simulink model "ackerman_ROS_neural_controller_v2"  (R2023a)
settings: Solver=FixedStepDiscrete  StartTime=0.0  StopTime=200  FixedStep=0.1  RelTol=1e-3
undefined symbols (not defined in the file or in its folder): Angular, Linear
libraries: neural x413, robotlib x15, robotcorelib x1
(part 10 of 17)

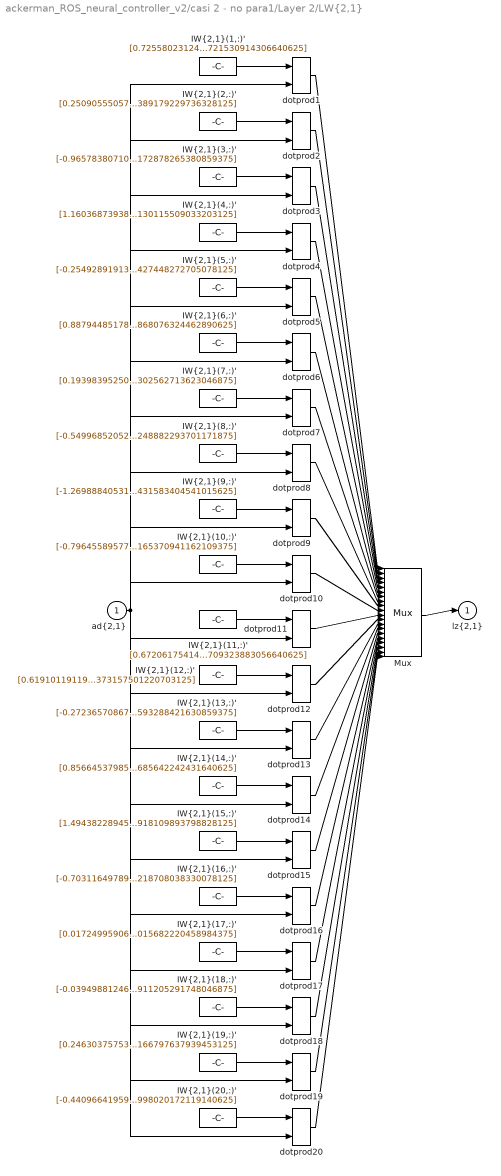
== system ackerman_ROS_neural_controller_v2/casi 2 - no para1/Layer 2/LW{2,1} ==
  "ad{2,1}" : Inport  PortDimensions=10  SampleTime=0.1
      mask Display: e = 0.06;c1 = [120 230 180]/255;c2 = ([120 230 180]+0)/(256+128);c3 = ([120 230 180]+128)/(256+128);patch([0 1 1 0],[0 0 1 1],c1);patch([0 1 1 1-e 1-e 0+e],[0 0 1 1-e 0+e 0+e],c2);patch([0 0 1 1-e 0+e 0+e],[0 1 1 1-e 1-e 0+e],c3);plot([0 1 1 0 0],[0 0 1 1 0]);
  "IW{2,1}(1,:)'" : Constant  Value=[0.7255802312437111822873703204095363616943359375;-0.959135021271336984938216119189746677875518798828125;0.292195933309013111678353880051872693002223968505859375;1.3155053067483366557866020229994319379329681396484375;-0.851881968454604621143744225264526903629302978515625;-1.0328524281587456723485729526146315038204193115234375;-0.2725914664811670551358702141442336142063140869140625;0.69933961328985816408021491952240467071533203125;-0.088878783625517987498909633359289728105068206787109375;-0.4504789263447295244446877404698170721530914306640625]
      mask Display: e = 0.06;c1 = [120 150 230]/255;c2 = ([120 150 230]+0)/383;c3 = ([120 150 230]+128)/383;patch([0 1 1 0],[0 0 1 1],c1);patch([0 1 1 1-e 1-e 0+e],[0 0 1 1-e 0+e 0+e],c2);patch([0 0 1 1-e 0+e 0+e],[0 1 1 1-e 1-e 0+e],c3);plot([0 1 1 0 0],[0 0 1 1 0]);disp('weights');
  "IW{2,1}(10,:)'" : Constant  Value=[-0.79645589577707454065347292271326296031475067138671875;0.255979770260327421649293455629958771169185638427734375;-0.258539951097875475571896686233230866491794586181640625;1.0207788991495245767282540327869355678558349609375;-0.24124933524105329762932115045259706676006317138671875;-0.72258293758172931209315947853610850870609283447265625;0.87006263229923608282234681610134430229663848876953125;-0.70559758504935310430283834648435004055500030517578125;-0.0123525145129407022681622407844770350493490695953369140625;-0.6747862752605688907436842782772146165370941162109375]
      mask Display: e = 0.06;c1 = [120 150 230]/255;c2 = ([120 150 230]+0)/383;c3 = ([120 150 230]+128)/383;patch([0 1 1 0],[0 0 1 1],c1);patch([0 1 1 1-e 1-e 0+e],[0 0 1 1-e 0+e 0+e],c2);patch([0 0 1 1-e 0+e 0+e],[0 1 1 1-e 1-e 0+e],c3);plot([0 1 1 0 0],[0 0 1 1 0]);disp('weights');
  "IW{2,1}(11,:)'" : Constant  Value=[0.67206175414446589488903782694251276552677154541015625;0.425012143990661284131959973819903098046779632568359375;-0.90070904319052724762428852045559324324131011962890625;-0.71047514245276188749045331860543228685855865478515625;0.62743503657371579862456201226450502872467041015625;-0.40397353982891914814246092646499164402484893798828125;0.1265477401734184381698611332467407919466495513916015625;-0.416411569496611011498288235088693909347057342529296875;0.0269578242680961095711911212902123224921524524688720703125;1.9286984680039014339314462631591595709323883056640625]
      mask Display: e = 0.06;c1 = [120 150 230]/255;c2 = ([120 150 230]+0)/383;c3 = ([120 150 230]+128)/383;patch([0 1 1 0],[0 0 1 1],c1);patch([0 1 1 1-e 1-e 0+e],[0 0 1 1-e 0+e 0+e],c2);patch([0 0 1 1-e 0+e 0+e],[0 1 1 1-e 1-e 0+e],c3);plot([0 1 1 0 0],[0 0 1 1 0]);disp('weights');
  "IW{2,1}(12,:)'" : Constant  Value=[0.61910119119551865196626749821007251739501953125;1.5566506758364762053048480083816684782505035400390625;0.007559785691830124727819129049066759762354195117950439453125;-0.2271652971788542807463073813778464682400226593017578125;-1.03507488578625395092558392207138240337371826171875;0.218995547321044925492827815105556510388851165771484375;0.257413353310532999618231997374095954000949859619140625;-0.09074896375455325514547411103194463066756725311279296875;0.51244231388938688009915267684846185147762298583984375;0.69550664112394511295889287794125266373157501220703125]
      mask Display: e = 0.06;c1 = [120 150 230]/255;c2 = ([120 150 230]+0)/383;c3 = ([120 150 230]+128)/383;patch([0 1 1 0],[0 0 1 1],c1);patch([0 1 1 1-e 1-e 0+e],[0 0 1 1-e 0+e 0+e],c2);patch([0 0 1 1-e 0+e 0+e],[0 1 1 1-e 1-e 0+e],c3);plot([0 1 1 0 0],[0 0 1 1 0]);disp('weights');
  "IW{2,1}(13,:)'" : Constant  Value=[-0.2723657086743267452533245887025259435176849365234375;0.51216475864015154062514056931831873953342437744140625;-1.0193552597301509532456975648528896272182464599609375;-1.1847191291297889392808428965508937835693359375;1.0773368660683753095241854680352844297885894775390625;0.0962534189837907228071145482317660935223102569580078125;-0.417721772937184265828136631171219050884246826171875;0.38947970915216412191028894085320644080638885498046875;0.337210418509659159980174081283621490001678466796875;0.220079813772727062026746125411591492593288421630859375]
      mask Display: e = 0.06;c1 = [120 150 230]/255;c2 = ([120 150 230]+0)/383;c3 = ([120 150 230]+128)/383;patch([0 1 1 0],[0 0 1 1],c1);patch([0 1 1 1-e 1-e 0+e],[0 0 1 1-e 0+e 0+e],c2);patch([0 0 1 1-e 0+e 0+e],[0 1 1 1-e 1-e 0+e],c3);plot([0 1 1 0 0],[0 0 1 1 0]);disp('weights');
  "IW{2,1}(14,:)'" : Constant  Value=[0.85664537985749278359293157336651347577571868896484375;0.56640828026000511474791210275725461542606353759765625;0.0140221107131337473228338552644345327280461788177490234375;0.2148298691543548966098597929885727353394031524658203125;-0.93403619601038467834541734191589057445526123046875;0.12856379595534705995163449188112281262874603271484375;-0.75467959982227217352601655875332653522491455078125;-0.63322516283317298313448873159359209239482879638671875;-1.0672216572169812565107349655590951442718505859375;-0.6144516641324175854066425017663277685642242431640625]
      mask Display: e = 0.06;c1 = [120 150 230]/255;c2 = ([120 150 230]+0)/383;c3 = ([120 150 230]+128)/383;patch([0 1 1 0],[0 0 1 1],c1);patch([0 1 1 1-e 1-e 0+e],[0 0 1 1-e 0+e 0+e],c2);patch([0 0 1 1-e 0+e 0+e],[0 1 1 1-e 1-e 0+e],c3);plot([0 1 1 0 0],[0 0 1 1 0]);disp('weights');
  "IW{2,1}(15,:)'" : Constant  Value=[1.494382289455435941505356822744943201541900634765625;-0.38028619508781480451631296091363765299320220947265625;-1.0111267060786659488513805627007968723773956298828125;-0.488055297640631380318154697306454181671142578125;0.3434831730449758868672915923525579273700714111328125;1.216268037924192579879445474944077432155609130859375;-0.1970804861360637982858889927229029126465320587158203125;-0.30493588644459268532926898842561058700084686279296875;1.429852600353733738103301220689900219440460205078125;0.55184388765904046625365708678145892918109893798828125]
      mask Display: e = 0.06;c1 = [120 150 230]/255;c2 = ([120 150 230]+0)/383;c3 = ([120 150 230]+128)/383;patch([0 1 1 0],[0 0 1 1],c1);patch([0 1 1 1-e 1-e 0+e],[0 0 1 1-e 0+e 0+e],c2);patch([0 0 1 1-e 0+e 0+e],[0 1 1 1-e 1-e 0+e],c3);plot([0 1 1 0 0],[0 0 1 1 0]);disp('weights');
  "IW{2,1}(16,:)'" : Constant  Value=[-0.70311649789439478741570610509370453655719757080078125;0.82719449320928128965846326536848209798336029052734375;0.52011078229624552182741581418667919933795928955078125;-0.7482339633582888449581105305696837604045867919921875;0.260733776152210439125411767236073501408100128173828125;1.257014055969282839697598319617100059986114501953125;0.514007980751157500520776011398993432521820068359375;0.06832775328143329829355678839419852010905742645263671875;1.355094864178037372681728811585344374179840087890625;0.58915716345959900923645591319655068218708038330078125]
      mask Display: e = 0.06;c1 = [120 150 230]/255;c2 = ([120 150 230]+0)/383;c3 = ([120 150 230]+128)/383;patch([0 1 1 0],[0 0 1 1],c1);patch([0 1 1 1-e 1-e 0+e],[0 0 1 1-e 0+e 0+e],c2);patch([0 0 1 1-e 0+e 0+e],[0 1 1 1-e 1-e 0+e],c3);plot([0 1 1 0 0],[0 0 1 1 0]);disp('weights');
  "IW{2,1}(17,:)'" : Constant  Value=[0.01724995906974446935322475837892852723598480224609375;-0.87370370646173001194512153233517892658710479736328125;1.02449594010034417124188621528446674346923828125;0.3546780425879723086524109021411277353763580322265625;0.5542510541573941740267628119909204542636871337890625;-1.519879697911841187618620097055099904537200927734375;1.9952410695173907750898933954886160790920257568359375;0.522496701742714453331473123398609459400177001953125;0.60216071280023564238348399157985113561153411865234375;1.3489645232526699114572465987293981015682220458984375]
      mask Display: e = 0.06;c1 = [120 150 230]/255;c2 = ([120 150 230]+0)/383;c3 = ([120 150 230]+128)/383;patch([0 1 1 0],[0 0 1 1],c1);patch([0 1 1 1-e 1-e 0+e],[0 0 1 1-e 0+e 0+e],c2);patch([0 0 1 1-e 0+e 0+e],[0 1 1 1-e 1-e 0+e],c3);plot([0 1 1 0 0],[0 0 1 1 0]);disp('weights');
  "IW{2,1}(18,:)'" : Constant  Value=[-0.039498812461870889956028207734561874531209468841552734375;0.458104116462539512344420700173941440880298614501953125;-0.12868703006185155945928499932051636278629302978515625;0.68295350186009751158877634225063957273960113525390625;-1.0871944340971875231360854741069488227367401123046875;-0.42803001209135571603070502533228136599063873291015625;0.012944291652409345427798825767240487039089202880859375;0.8094050995384247659814036524039693176746368408203125;-0.562292589961300048884140778682194650173187255859375;0.1292007200127660293542675162825617007911205291748046875]
      mask Display: e = 0.06;c1 = [120 150 230]/255;c2 = ([120 150 230]+0)/383;c3 = ([120 150 230]+128)/383;patch([0 1 1 0],[0 0 1 1],c1);patch([0 1 1 1-e 1-e 0+e],[0 0 1 1-e 0+e 0+e],c2);patch([0 0 1 1-e 0+e 0+e],[0 1 1 1-e 1-e 0+e],c3);plot([0 1 1 0 0],[0 0 1 1 0]);disp('weights');
  "IW{2,1}(19,:)'" : Constant  Value=[0.2463037575343004770278554360629641450941562652587890625;1.082908833346408528086612932384014129638671875;-0.5431543815046693257642118624062277376651763916015625;1.2737764365786403697455853034625761210918426513671875;0.543977471682644431183462074841372668743133544921875;-0.85893985210927337181630036866408772766590118408203125;1.871626995457029263292270115925930440425872802734375;0.0825784829680522580730439585749991238117218017578125;-1.654760344583033226939505766495130956172943115234375;0.2404324935540936014621848926253733225166797637939453125]
      mask Display: e = 0.06;c1 = [120 150 230]/255;c2 = ([120 150 230]+0)/383;c3 = ([120 150 230]+128)/383;patch([0 1 1 0],[0 0 1 1],c1);patch([0 1 1 1-e 1-e 0+e],[0 0 1 1-e 0+e 0+e],c2);patch([0 0 1 1-e 0+e 0+e],[0 1 1 1-e 1-e 0+e],c3);plot([0 1 1 0 0],[0 0 1 1 0]);disp('weights');
  "IW{2,1}(2,:)'" : Constant  Value=[0.2509055505702744159890471564722247421741485595703125;-1.25881579798349463317208574153482913970947265625;1.33862512869737404486158993677236139774322509765625;0.315714701756230564644312153177452273666858673095703125;-1.2366679233488728772982767623034305870532989501953125;0.3493751303882339787065802738652564585208892822265625;0.01409598964836229935404521285136070218868553638458251953125;1.27609628826768695120108532137237489223480224609375;-0.1335788420752038463401589751811116002500057220458984375;-0.93661901416684145704749653305043466389179229736328125]
      mask Display: e = 0.06;c1 = [120 150 230]/255;c2 = ([120 150 230]+0)/383;c3 = ([120 150 230]+128)/383;patch([0 1 1 0],[0 0 1 1],c1);patch([0 1 1 1-e 1-e 0+e],[0 0 1 1-e 0+e 0+e],c2);patch([0 0 1 1-e 0+e 0+e],[0 1 1 1-e 1-e 0+e],c3);plot([0 1 1 0 0],[0 0 1 1 0]);disp('weights');
  "IW{2,1}(20,:)'" : Constant  Value=[-0.44096641959653981590605553719797171652317047119140625;0.7083902543346669578028240721323527395725250244140625;-0.5166341286167612789625991354114376008510589599609375;0.9049323980779118148376483077299781143665313720703125;-1.271794249096482420924303369247354567050933837890625;-0.68138595653020306297520392035949043929576873779296875;-0.90212325864638021055696981420624069869518280029296875;-0.45820526458276022996329857051023282110691070556640625;-0.020846715917271947671185472472643596120178699493408203125;-0.68369139124353583980564508237875998020172119140625]
      mask Display: e = 0.06;c1 = [120 150 230]/255;c2 = ([120 150 230]+0)/383;c3 = ([120 150 230]+128)/383;patch([0 1 1 0],[0 0 1 1],c1);patch([0 1 1 1-e 1-e 0+e],[0 0 1 1-e 0+e 0+e],c2);patch([0 0 1 1-e 0+e 0+e],[0 1 1 1-e 1-e 0+e],c3);plot([0 1 1 0 0],[0 0 1 1 0]);disp('weights');
  "IW{2,1}(3,:)'" : Constant  Value=[-0.9657838071053219675121681575546972453594207763671875;-0.29459222518749650365776915350579656660556793212890625;-0.9657645759044359845546523501980118453502655029296875;0.472664168879096069364464938189485110342502593994140625;-0.4647204412011516350133888408890925347805023193359375;0.0489842324695661524014411725147510878741741180419921875;-0.470447392631997807210808559830184094607830047607421875;-0.75556461890030190975409141174168325960636138916015625;-0.77960517042681154453731551257078535854816436767578125;0.1635230428322337059565683148321113549172878265380859375]
      mask Display: e = 0.06;c1 = [120 150 230]/255;c2 = ([120 150 230]+0)/383;c3 = ([120 150 230]+128)/383;patch([0 1 1 0],[0 0 1 1],c1);patch([0 1 1 1-e 1-e 0+e],[0 0 1 1-e 0+e 0+e],c2);patch([0 0 1 1-e 0+e 0+e],[0 1 1 1-e 1-e 0+e],c3);plot([0 1 1 0 0],[0 0 1 1 0]);disp('weights');
  "IW{2,1}(4,:)'" : Constant  Value=[1.1603687393829453800009332553599961102008819580078125;-0.43444035743057363152530570005183108150959014892578125;-0.2327820794505396639895167254508123733103275299072265625;1.0752460303334367974770202636136673390865325927734375;0.0409481506539224049401326510633225552737712860107421875;-0.52422297129341666188651061020209453999996185302734375;0.97732432532743407360698029151535592973232269287109375;1.670364407889719959854346598149277269840240478515625;-0.57438837959386257470129066859954036772251129150390625;0.06045821031614935503473162725640577264130115509033203125]
      mask Display: e = 0.06;c1 = [120 150 230]/255;c2 = ([120 150 230]+0)/383;c3 = ([120 150 230]+128)/383;patch([0 1 1 0],[0 0 1 1],c1);patch([0 1 1 1-e 1-e 0+e],[0 0 1 1-e 0+e 0+e],c2);patch([0 0 1 1-e 0+e 0+e],[0 1 1 1-e 1-e 0+e],c3);plot([0 1 1 0 0],[0 0 1 1 0]);disp('weights');
  "IW{2,1}(5,:)'" : Constant  Value=[-0.254928919131068576486853771712048910558223724365234375;0.73622325216995931906893702034722082316875457763671875;-0.2115569379132722083181050720668281428515911102294921875;0.16011668696643288622993850367492996156215667724609375;-1.007294432717205978633501217700541019439697265625;0.879084198460805765762415830977261066436767578125;0.57105308322778036700384518553619273006916046142578125;-0.1648122755865679411879654026051866821944713592529296875;0.9415158413094939504617286729626357555389404296875;0.525759644457871377909441434894688427448272705078125]
      mask Display: e = 0.06;c1 = [120 150 230]/255;c2 = ([120 150 230]+0)/383;c3 = ([120 150 230]+128)/383;patch([0 1 1 0],[0 0 1 1],c1);patch([0 1 1 1-e 1-e 0+e],[0 0 1 1-e 0+e 0+e],c2);patch([0 0 1 1-e 0+e 0+e],[0 1 1 1-e 1-e 0+e],c3);plot([0 1 1 0 0],[0 0 1 1 0]);disp('weights');
  "IW{2,1}(6,:)'" : Constant  Value=[0.88794485178955573356773811610764823853969573974609375;0.2324274258381906488324375459342263638973236083984375;0.858625944853660172384479665197432041168212890625;-0.79953285474529989240721761234453879296779632568359375;0.3246840807043895882344486381043680012226104736328125;0.70300148951327512403253194861463271081447601318359375;0.72709749834294801207335012804833240807056427001953125;-0.059841883781344189230377850208242307417094707489013671875;0.55259353871622185483403200123575516045093536376953125;0.303105422786621725439459851259016431868076324462890625]
      mask Display: e = 0.06;c1 = [120 150 230]/255;c2 = ([120 150 230]+0)/383;c3 = ([120 150 230]+128)/383;patch([0 1 1 0],[0 0 1 1],c1);patch([0 1 1 1-e 1-e 0+e],[0 0 1 1-e 0+e 0+e],c2);patch([0 0 1 1-e 0+e 0+e],[0 1 1 1-e 1-e 0+e],c3);plot([0 1 1 0 0],[0 0 1 1 0]);disp('weights');
  "IW{2,1}(7,:)'" : Constant  Value=[0.19398395250211120099947947892360389232635498046875;0.1806780802861871204623156472734990529716014862060546875;1.06574239323498431986081413924694061279296875;-0.17040549486612699414678218090557493269443511962890625;0.89158393834403704136803980873082764446735382080078125;-1.4919986389830948159129775376641191542148590087890625;-0.69437571656851115875497271190397441387176513671875;0.75295094637079718058458865925786085426807403564453125;-0.8595816234580855308422542293556034564971923828125;0.384089854587841894595356961872312240302562713623046875]
      mask Display: e = 0.06;c1 = [120 150 230]/255;c2 = ([120 150 230]+0)/383;c3 = ([120 150 230]+128)/383;patch([0 1 1 0],[0 0 1 1],c1);patch([0 1 1 1-e 1-e 0+e],[0 0 1 1-e 0+e 0+e],c2);patch([0 0 1 1-e 0+e 0+e],[0 1 1 1-e 1-e 0+e],c3);plot([0 1 1 0 0],[0 0 1 1 0]);disp('weights');
  "IW{2,1}(8,:)'" : Constant  Value=[-0.5499685205288944445101151359267532825469970703125;1.32755393052571424306051994790323078632354736328125;0.551262479059708265793915415997616946697235107421875;-0.406055752844285688940573209038120694458484649658203125;0.311009629150236277528307482498348690569400787353515625;-1.5072835912126902879748513441882096230983734130859375;0.955100302665503164689653203822672367095947265625;0.1511551582338540866690124175875098444521427154541015625;-0.351323789684884868478320640861056745052337646484375;-0.54768695672100065063858664871077053248882293701171875]
      mask Display: e = 0.06;c1 = [120 150 230]/255;c2 = ([120 150 230]+0)/383;c3 = ([120 150 230]+128)/383;patch([0 1 1 0],[0 0 1 1],c1);patch([0 1 1 1-e 1-e 0+e],[0 0 1 1-e 0+e 0+e],c2);patch([0 0 1 1-e 0+e 0+e],[0 1 1 1-e 1-e 0+e],c3);plot([0 1 1 0 0],[0 0 1 1 0]);disp('weights');
  "IW{2,1}(9,:)'" : Constant  Value=[-1.2698884053102796887202430298202671110630035400390625;1.157998294185372145648216246627271175384521484375;0.8644080951922508138096645780024118721485137939453125;-0.082862245337413986678853916600928641855716705322265625;-0.003908380542946330617193329004521729075349867343902587890625;0.98242726341600217221383672949741594493389129638671875;0.61596730978288605218295970189501531422138214111328125;0.96021102700887361880432990801637060940265655517578125;0.98543515097618972209403409578953869640827178955078125;-0.16275623645196957145486749141127802431583404541015625]
      mask Display: e = 0.06;c1 = [120 150 230]/255;c2 = ([120 150 230]+0)/383;c3 = ([120 150 230]+128)/383;patch([0 1 1 0],[0 0 1 1],c1);patch([0 1 1 1-e 1-e 0+e],[0 0 1 1-e 0+e 0+e],c2);patch([0 0 1 1-e 0+e 0+e],[0 1 1 1-e 1-e 0+e],c3);plot([0 1 1 0 0],[0 0 1 1 0]);disp('weights');
  Mux : Mux  Inputs=20
      mask Display: e = 0.06;c1 = [120 150 230]/255;c2 = ([120 150 230]+0)/383;c3 = ([120 150 230]+128)/383;patch([0 1 1 0],[0 0 1 1],c1);patch([0 1 1 1-e 1-e 0+e],[0 0 1 1-e 0+e 0+e],c2);patch([0 0 1 1-e 0+e 0+e],[0 1 1 1-e 1-e 0+e],c3);plot([0 1 1 0 0],[0 0 1 1 0]);disp('Mux');
  dotprod{1..20} (20 alike) : neural/Weight Functions/dotprod
  "lz{2,1}" : Outport
      mask Display: e = 0.06;c1 = [120 230 180]/255;c2 = ([120 230 180]+0)/(256+128);c3 = ([120 230 180]+128)/(256+128);patch([0 1 1 0],[0 0 1 1],c1);patch([0 1 1 1-e 1-e 0+e],[0 0 1 1-e 0+e 0+e],c2);patch([0 0 1 1-e 0+e 0+e],[0 1 1 1-e 1-e 0+e],c3);plot([0 1 1 0 0],[0 0 1 1 0]);
  wires:
  "IW{2,1}(1,:)'"/1 -> dotprod1/1
  "ad{2,1}"/1 -> dotprod1/2, dotprod2/2, dotprod3/2, dotprod4/2, dotprod5/2, dotprod6/2, dotprod7/2, dotprod8/2, dotprod9/2, dotprod10/2, dotprod11/2, dotprod12/2, dotprod13/2, dotprod14/2, dotprod15/2, dotprod16/2, dotprod17/2, dotprod18/2, dotprod19/2, dotprod20/2
  dotprod1/1 -> Mux/1
  "IW{2,1}(2,:)'"/1 -> dotprod2/1
  dotprod2/1 -> Mux/2
  "IW{2,1}(3,:)'"/1 -> dotprod3/1
  dotprod3/1 -> Mux/3
  "IW{2,1}(4,:)'"/1 -> dotprod4/1
  dotprod4/1 -> Mux/4
  "IW{2,1}(5,:)'"/1 -> dotprod5/1
  dotprod5/1 -> Mux/5
  "IW{2,1}(6,:)'"/1 -> dotprod6/1
  dotprod6/1 -> Mux/6
  "IW{2,1}(7,:)'"/1 -> dotprod7/1
  dotprod7/1 -> Mux/7
  "IW{2,1}(8,:)'"/1 -> dotprod8/1
  dotprod8/1 -> Mux/8
  "IW{2,1}(9,:)'"/1 -> dotprod9/1
  dotprod9/1 -> Mux/9
  "IW{2,1}(10,:)'"/1 -> dotprod10/1
  dotprod10/1 -> Mux/10
  "IW{2,1}(11,:)'"/1 -> dotprod11/1
  dotprod11/1 -> Mux/11
  "IW{2,1}(12,:)'"/1 -> dotprod12/1
  dotprod12/1 -> Mux/12
  "IW{2,1}(13,:)'"/1 -> dotprod13/1
  dotprod13/1 -> Mux/13
  "IW{2,1}(14,:)'"/1 -> dotprod14/1
  dotprod14/1 -> Mux/14
  "IW{2,1}(15,:)'"/1 -> dotprod15/1
  dotprod15/1 -> Mux/15
  "IW{2,1}(16,:)'"/1 -> dotprod16/1
  dotprod16/1 -> Mux/16
  "IW{2,1}(17,:)'"/1 -> dotprod17/1
  dotprod17/1 -> Mux/17
  "IW{2,1}(18,:)'"/1 -> dotprod18/1
  dotprod18/1 -> Mux/18
  "IW{2,1}(19,:)'"/1 -> dotprod19/1
  dotprod19/1 -> Mux/19
  "IW{2,1}(20,:)'"/1 -> dotprod20/1
  dotprod20/1 -> Mux/20
  Mux/1 -> "lz{2,1}"/1

== system ackerman_ROS_neural_controller_v2/casi 2 - no para1/Layer 3/Delays 1 ==
  "p{3}" : Inport  PortDimensions=20  SampleTime=0.1
      mask Display: e = 0.06;c1 = [120 230 180]/255;c2 = ([120 230 180]+0)/(256+128);c3 = ([120 230 180]+128)/(256+128);patch([0 1 1 0],[0 0 1 1],c1);patch([0 1 1 1-e 1-e 0+e],[0 0 1 1-e 0+e 0+e],c2);patch([0 0 1 1-e 0+e 0+e],[0 1 1 1-e 1-e 0+e],c3);plot([0 1 1 0 0],[0 0 1 1 0]);
  mux : Mux  Inputs=1
      mask Display: e = 0.06;c1 = [120 150 230]/255;c2 = ([120 150 230]+0)/383;c3 = ([120 150 230]+128)/383;patch([0 1 1 0],[0 0 1 1],c1);patch([0 1 1 1-e 1-e 0+e],[0 0 1 1-e 0+e 0+e],c2);patch([0 0 1 1-e 0+e 0+e],[0 1 1 1-e 1-e 0+e],c3);plot([0 1 1 0 0],[0 0 1 1 0]);disp('Mux')
  "pd{3,2}" : Outport
      mask Display: e = 0.06;c1 = [120 230 180]/255;c2 = ([120 230 180]+0)/(256+128);c3 = ([120 230 180]+128)/(256+128);patch([0 1 1 0],[0 0 1 1],c1);patch([0 1 1 1-e 1-e 0+e],[0 0 1 1-e 0+e 0+e],c2);patch([0 0 1 1-e 0+e 0+e],[0 1 1 1-e 1-e 0+e],c3);plot([0 1 1 0 0],[0 0 1 1 0]);
  wires:
  "p{3}"/1 -> mux/1
  mux/1 -> "pd{3,2}"/1

== system ackerman_ROS_neural_controller_v2/casi 2 - no para1/Layer 3/LW{3,2} ==
  "ad{3,2}" : Inport  PortDimensions=20  SampleTime=0.1
      mask Display: e = 0.06;c1 = [120 230 180]/255;c2 = ([120 230 180]+0)/(256+128);c3 = ([120 230 180]+128)/(256+128);patch([0 1 1 0],[0 0 1 1],c1);patch([0 1 1 1-e 1-e 0+e],[0 0 1 1-e 0+e 0+e],c2);patch([0 0 1 1-e 0+e 0+e],[0 1 1 1-e 1-e 0+e],c3);plot([0 1 1 0 0],[0 0 1 1 0]);
  "IW{3,2}(1,:)'" : Constant  Value=[-0.0484176990196327483584326500931638292968273162841796875;-0.395379687388352107912936617140076123178005218505859375;0.393415072911054541915376603355980478227138519287109375;-1.038674743874415273836575579480268061161041259765625;0.347480719944031124502004104215302504599094390869140625;0.06059305762399079531288492717067128978669643402099609375;0.2875916208848394717279006727039813995361328125;0.09194192813162926913861383582116104662418365478515625;0.53487908914414028505035503258113749325275421142578125;-0.382680366310746311597767999046482145786285400390625;-0.8979087999904862282818385210703127086162567138671875;0.65522685922687184945090166365844197571277618408203125;0.5095776020782187831770215780124999582767486572265625;-0.197085087087855936882618834715685807168483734130859375;0.25153060920636038932940437007346190512180328369140625;-0.611258303462508312264844789751805365085601806640625;-0.427149502993451168908478621233371086418628692626953125;0.420627131398296494335653505913796834647655487060546875;0.225811354993810609048665583031834103167057037353515625;0.049771356479713195486436205783320474438369274139404296875]
      mask Display: e = 0.06;c1 = [120 150 230]/255;c2 = ([120 150 230]+0)/383;c3 = ([120 150 230]+128)/383;patch([0 1 1 0],[0 0 1 1],c1);patch([0 1 1 1-e 1-e 0+e],[0 0 1 1-e 0+e 0+e],c2);patch([0 0 1 1-e 0+e 0+e],[0 1 1 1-e 1-e 0+e],c3);plot([0 1 1 0 0],[0 0 1 1 0]);disp('weights');
  "IW{3,2}(10,:)'" : Constant  Value=[-0.01368126341638766819974737387610730365850031375885009765625;0.504490183492814825427785763167776167392730712890625;0.426031002353343513089356520140427164733409881591796875;-0.435042693782689171566602226448594592511653900146484375;0.881139928749048007006194893619976937770843505859375;0.4696792355255043904804779231199063360691070556640625;-0.08656168531149317779682661466722493059933185577392578125;-0.8781220485159104693906328975572250783443450927734375;0.44758265796058982477489962548133917152881622314453125;-0.27772691487725331693781072317506186664104461669921875;0.229381788105754769180322227839496918022632598876953125;-0.5446755626299866204220734289265237748622894287109375;0.3211232937139707477314232164644636213779449462890625;0.448702108190841941759430255842744372785091400146484375;0.331797807801021027440668831332004629075527191162109375;-0.498265268757341173166963699259213171899318695068359375;-0.23411347435325746690892856349819339811801910400390625;0.0210578720712033366779802889823258738033473491668701171875;-0.2415552036546391445615000748148304410278797149658203125;0.140035878595142937452777687212801538407802581787109375]
      mask Display: e = 0.06;c1 = [120 150 230]/255;c2 = ([120 150 230]+0)/383;c3 = ([120 150 230]+128)/383;patch([0 1 1 0],[0 0 1 1],c1);patch([0 1 1 1-e 1-e 0+e],[0 0 1 1-e 0+e 0+e],c2);patch([0 0 1 1-e 0+e 0+e],[0 1 1 1-e 1-e 0+e],c3);plot([0 1 1 0 0],[0 0 1 1 0]);disp('weights');
  "IW{3,2}(2,:)'" : Constant  Value=[0.56494013059803827037086421114508993923664093017578125;0.7078203097826136769299409934319555759429931640625;0.000457193189375819223664587642730339211993850767612457275390625;0.638713459938562433393371975398622453212738037109375;-0.069241917769923222447658872624742798507213592529296875;-0.449108257291477797057410725756199099123477935791015625;-0.53053658786290480708913719354313798248767852783203125;0.780176911754975943580348030081950128078460693359375;-1.6311746611531905415404253290034830570220947265625;0.37912911732154530586313967432943172752857208251953125;-0.382805627167483841777340103362803347408771514892578125;-0.53198531883968269706741693880758248269557952880859375;0.061789076449593881290578423204351565800607204437255859375;-0.65539716169900741338238958633155561983585357666015625;-0.11352510936119238060815206381448660977184772491455078125;1.5250382906488493262031624908559024333953857421875;1.601284278105115976842398595181293785572052001953125;-0.08400375505645678309019075413743848912417888641357421875;2.155330647951852807153727553668431937694549560546875;-1.1592881276125990286374189963680692017078399658203125]
      mask Display: e = 0.06;c1 = [120 150 230]/255;c2 = ([120 150 230]+0)/383;c3 = ([120 150 230]+128)/383;patch([0 1 1 0],[0 0 1 1],c1);patch([0 1 1 1-e 1-e 0+e],[0 0 1 1-e 0+e 0+e],c2);patch([0 0 1 1-e 0+e 0+e],[0 1 1 1-e 1-e 0+e],c3);plot([0 1 1 0 0],[0 0 1 1 0]);disp('weights');
  "IW{3,2}(3,:)'" : Constant  Value=[0.60895054427480099779046440744423307478427886962890625;0.2335767631510164699104592500589205883443355560302734375;-0.30883277163937294940154743017046712338924407958984375;-0.1877304673004198398711395157079095952212810516357421875;-0.29079185160617926353410211959271691739559173583984375;-0.304067793021201626668670314757036976516246795654296875;-0.284412193752655306777654686811729334294795989990234375;0.08798429174072987246635335623068385757505893707275390625;-0.896348748846316656369026532047428190708160400390625;-0.132676383501228400962901332604815252125263214111328125;0.606235265517712118565896162181161344051361083984375;-0.317064170117056398634503011635388247668743133544921875;-0.23840321210247450434138727359822951257228851318359375;-0.173841524963109395063298734385170973837375640869140625;1.2828124600645056663239529370912350714206695556640625;0.276103327176183854785307403290062211453914642333984375;-1.13344204103107326631061368971131742000579833984375;-0.13628110175208563159543473375379107892513275146484375;-0.34442818809230202337090531727881170809268951416015625;-0.447265541040587744081591381473117507994174957275390625]
      mask Display: e = 0.06;c1 = [120 150 230]/255;c2 = ([120 150 230]+0)/383;c3 = ([120 150 230]+128)/383;patch([0 1 1 0],[0 0 1 1],c1);patch([0 1 1 1-e 1-e 0+e],[0 0 1 1-e 0+e 0+e],c2);patch([0 0 1 1-e 0+e 0+e],[0 1 1 1-e 1-e 0+e],c3);plot([0 1 1 0 0],[0 0 1 1 0]);disp('weights');
  "IW{3,2}(4,:)'" : Constant  Value=[-0.250612074616448798902723638093448244035243988037109375;0.63265614505663136934998647120664827525615692138671875;-0.411246666155860751690198640062590129673480987548828125;0.03314326526697299046819722434520372189581394195556640625;-0.543020000350967535496238269843161106109619140625;0.0082818796179317498429295341111355810426175594329833984375;-0.316304460057695024932655769589473493397235870361328125;-0.49312817946492082388232347511802799999713897705078125;0.048611114881914212204616632106990437023341655731201171875;-0.1999078084624461570939502053079195320606231689453125;-1.225739614370188856895538265234790742397308349609375;0.1629612879460799190756148391301394440233707427978515625;-0.1863913385074375261840629036669270135462284088134765625;0.56730333251757436574536086482112295925617218017578125;-0.10423588589274364324399613224159111268818378448486328125;-0.2268633967236502735342895675785257481038570404052734375;0.1308941704119328253153042851408827118575572967529296875;-0.09124899775299695481312056699607637710869312286376953125;0.18680493454028590516458052661619149148464202880859375;-0.26895471036517959451117576463730074465274810791015625]
      mask Display: e = 0.06;c1 = [120 150 230]/255;c2 = ([120 150 230]+0)/383;c3 = ([120 150 230]+128)/383;patch([0 1 1 0],[0 0 1 1],c1);patch([0 1 1 1-e 1-e 0+e],[0 0 1 1-e 0+e 0+e],c2);patch([0 0 1 1-e 0+e 0+e],[0 1 1 1-e 1-e 0+e],c3);plot([0 1 1 0 0],[0 0 1 1 0]);disp('weights');
  "IW{3,2}(5,:)'" : Constant  Value=[0.052541964412058113353953814339547534473240375518798828125;0.0139732893035238135703846040769349201582372188568115234375;0.437897012575633237663197405709070153534412384033203125;0.894632899542399773196166279376484453678131103515625;-0.050453205431981902606697332203111727721989154815673828125;0.07387656323479947773069653749189455993473529815673828125;-0.354682182158403136451596537881414406001567840576171875;-0.39884021545097281258307475582114420831203460693359375;-0.477720893427135140374417687780805863440036773681640625;1.11406579409307493477854222874157130718231201171875;0.361010401542299519395129436816205270588397979736328125;-0.795725538351665928615830125636421144008636474609375;0.74789040355670211024374793851166032254695892333984375;0.356255389846889369831473004524013958871364593505859375;0.45454901901046229628633454922237433493137359619140625;-0.50929240554063015533614589003263972699642181396484375;0.331498327896553146576508197540533728897571563720703125;0.263872979231392024157543119144975207746028900146484375;0.43743423503859435452767456808942370116710662841796875;-0.67381113487006860651717943255789577960968017578125]
      mask Display: e = 0.06;c1 = [120 150 230]/255;c2 = ([120 150 230]+0)/383;c3 = ([120 150 230]+128)/383;patch([0 1 1 0],[0 0 1 1],c1);patch([0 1 1 1-e 1-e 0+e],[0 0 1 1-e 0+e 0+e],c2);patch([0 0 1 1-e 0+e 0+e],[0 1 1 1-e 1-e 0+e],c3);plot([0 1 1 0 0],[0 0 1 1 0]);disp('weights');
  "IW{3,2}(6,:)'" : Constant  Value=[-0.717852651845437339517275177058763802051544189453125;-1.28235954231634963207397959195077419281005859375;-0.1408553837144228271238688421362894587218761444091796875;-0.9076476327916795927563953227945603430271148681640625;0.434787414091763080303820743210962973535060882568359375;-0.472539307864701052519507129545672796666622161865234375;0.80970930118478123826974979238002561032772064208984375;0.2214618295449891360870964263085625134408473968505859375;0.125029750047555399117271690556663088500499725341796875;0.252669480912385002735476291491067968308925628662109375;0.311213249656233370554758721482357941567897796630859375;-0.45547944680093210845228668404160998761653900146484375;0.177534239954488637369678372124326415359973907470703125;0.040073510097663529727629594390236889012157917022705078125;0.5401306610468126212509787364979274570941925048828125;0.399421861018017521072209774501970969140529632568359375;-0.79132623911901933677626175267505459487438201904296875;0.7286661469225170773000854751444421708583831787109375;0.032126227051297286119169172025067382492125034332275390625;-0.0702748654542214856721926707905367948114871978759765625]
      mask Display: e = 0.06;c1 = [120 150 230]/255;c2 = ([120 150 230]+0)/383;c3 = ([120 150 230]+128)/383;patch([0 1 1 0],[0 0 1 1],c1);patch([0 1 1 1-e 1-e 0+e],[0 0 1 1-e 0+e 0+e],c2);patch([0 0 1 1-e 0+e 0+e],[0 1 1 1-e 1-e 0+e],c3);plot([0 1 1 0 0],[0 0 1 1 0]);disp('weights');
  "IW{3,2}(7,:)'" : Constant  Value=[0.450744663975816639567284482836839742958545684814453125;0.6791813046995789360238404697156511247158050537109375;-0.194046682628332523012915089566376991569995880126953125;-0.451728390550129199620954523197724483907222747802734375;-0.19671452843368675278412638363079167902469635009765625;0.217206612761508599529491903012967668473720550537109375;-1.004438195645815934398115132353268563747406005859375;0.21224892787992555298615116043947637081146240234375;-0.21004589760710656864972634139121510088443756103515625;-0.48051675558990603054354551204596646130084991455078125;0.97468753125278573268275295049534179270267486572265625;1.252085813979519901550929716904647648334503173828125;0.68436181197922885122153502379660494625568389892578125;-0.17646605656571845432978307144367136061191558837890625;0.45706076188125710491050313066807575523853302001953125;-0.034509688525754589338845335078076459467411041259765625;0.5800994374669363740082417280063964426517486572265625;-0.234615294919385097838215870069689117372035980224609375;-1.137915917216942407463875497342087328433990478515625;-0.2174470872481620575822347518624155782163143157958984375]
      mask Display: e = 0.06;c1 = [120 150 230]/255;c2 = ([120 150 230]+0)/383;c3 = ([120 150 230]+128)/383;patch([0 1 1 0],[0 0 1 1],c1);patch([0 1 1 1-e 1-e 0+e],[0 0 1 1-e 0+e 0+e],c2);patch([0 0 1 1-e 0+e 0+e],[0 1 1 1-e 1-e 0+e],c3);plot([0 1 1 0 0],[0 0 1 1 0]);disp('weights');
  "IW{3,2}(8,:)'" : Constant  Value=[-0.21668321620218089496034963303827680647373199462890625;-0.3245942951988920466277477316907607018947601318359375;0.12070929362761638470313840798553428612649440765380859375;-0.1666565068043235620098840854552690871059894561767578125;-0.49969049046460523033630352074396796524524688720703125;0.52305469737378940120464676510891877114772796630859375;-0.2468409618021104312557412185924476943910121917724609375;0.73930547176299576950242453676764853298664093017578125;-0.57293450482219709929410100812674500048160552978515625;-0.2428764701009196169678716614725999534130096435546875;0.32881792990538782905929338085115887224674224853515625;0.36325934661455760998904906955431215465068817138671875;0.7922326663627570209058603722951374948024749755859375;-0.20167865314024713274676514629391022026538848876953125;-0.2026029815600232375505385107317124493420124053955078125;0.2018166897190335762335422487012692727148532867431640625;0.0031200586844526731304660938093320510233752429485321044921875;0.0251437474744682087912650558791938237845897674560546875;0.5779109539692142138989083832711912691593170166015625;0.352521086162789043516596620975178666412830352783203125]
      mask Display: e = 0.06;c1 = [120 150 230]/255;c2 = ([120 150 230]+0)/383;c3 = ([120 150 230]+128)/383;patch([0 1 1 0],[0 0 1 1],c1);patch([0 1 1 1-e 1-e 0+e],[0 0 1 1-e 0+e 0+e],c2);patch([0 0 1 1-e 0+e 0+e],[0 1 1 1-e 1-e 0+e],c3);plot([0 1 1 0 0],[0 0 1 1 0]);disp('weights');
  "IW{3,2}(9,:)'" : Constant  Value=[0.34054563485466093908371476572938263416290283203125;-0.401153378983528263734825713981990702450275421142578125;0.5791311694308640678485744501813314855098724365234375;1.20624482859577764060077242902480065822601318359375;0.275013800902427718586551463886280544102191925048828125;-0.1771102374271899815294517566144349984824657440185546875;0.12519477305321402571536282266606576740741729736328125;0.310156653036746166041126571144559420645236968994140625;-0.06723019498821179718017759796566679142415523529052734375;-0.24898597257160937079589757559006102383136749267578125;0.2352107285989128160341721240911283530294895172119140625;-0.1379816630619636053101118022823357023298740386962890625;0.294189276011052935899670046637766063213348388671875;-0.1031329747589122269868511239110375754535198211669921875;0.9098051480875855023811027422198094427585601806640625;-0.61804610644610613601201976052834652364253997802734375;0.65371172651814968279637696468853391706943511962890625;-0.042369338077858344215886887695887708105146884918212890625;0.08756867467303543206558202882661134935915470123291015625;-1.137602951954017616031933357589878141880035400390625]
      mask Display: e = 0.06;c1 = [120 150 230]/255;c2 = ([120 150 230]+0)/383;c3 = ([120 150 230]+128)/383;patch([0 1 1 0],[0 0 1 1],c1);patch([0 1 1 1-e 1-e 0+e],[0 0 1 1-e 0+e 0+e],c2);patch([0 0 1 1-e 0+e 0+e],[0 1 1 1-e 1-e 0+e],c3);plot([0 1 1 0 0],[0 0 1 1 0]);disp('weights');
  Mux : Mux  Inputs=10
      mask Display: e = 0.06;c1 = [120 150 230]/255;c2 = ([120 150 230]+0)/383;c3 = ([120 150 230]+128)/383;patch([0 1 1 0],[0 0 1 1],c1);patch([0 1 1 1-e 1-e 0+e],[0 0 1 1-e 0+e 0+e],c2);patch([0 0 1 1-e 0+e 0+e],[0 1 1 1-e 1-e 0+e],c3);plot([0 1 1 0 0],[0 0 1 1 0]);disp('Mux');
  dotprod{1..10} (10 alike) : neural/Weight Functions/dotprod
  "lz{3,2}" : Outport
      mask Display: e = 0.06;c1 = [120 230 180]/255;c2 = ([120 230 180]+0)/(256+128);c3 = ([120 230 180]+128)/(256+128);patch([0 1 1 0],[0 0 1 1],c1);patch([0 1 1 1-e 1-e 0+e],[0 0 1 1-e 0+e 0+e],c2);patch([0 0 1 1-e 0+e 0+e],[0 1 1 1-e 1-e 0+e],c3);plot([0 1 1 0 0],[0 0 1 1 0]);
  wires:
  "IW{3,2}(1,:)'"/1 -> dotprod1/1
  "ad{3,2}"/1 -> dotprod1/2, dotprod2/2, dotprod3/2, dotprod4/2, dotprod5/2, dotprod6/2, dotprod7/2, dotprod8/2, dotprod9/2, dotprod10/2
  dotprod1/1 -> Mux/1
  "IW{3,2}(2,:)'"/1 -> dotprod2/1
  dotprod2/1 -> Mux/2
  "IW{3,2}(3,:)'"/1 -> dotprod3/1
  dotprod3/1 -> Mux/3
  "IW{3,2}(4,:)'"/1 -> dotprod4/1
  dotprod4/1 -> Mux/4
  "IW{3,2}(5,:)'"/1 -> dotprod5/1
  dotprod5/1 -> Mux/5
  "IW{3,2}(6,:)'"/1 -> dotprod6/1
  dotprod6/1 -> Mux/6
  "IW{3,2}(7,:)'"/1 -> dotprod7/1
  dotprod7/1 -> Mux/7
  "IW{3,2}(8,:)'"/1 -> dotprod8/1
  dotprod8/1 -> Mux/8
  "IW{3,2}(9,:)'"/1 -> dotprod9/1
  dotprod9/1 -> Mux/9
  "IW{3,2}(10,:)'"/1 -> dotprod10/1
  dotprod10/1 -> Mux/10
  Mux/1 -> "lz{3,2}"/1

== system ackerman_ROS_neural_controller_v2/casi 2 - no para1/Layer 4/Delays 1 ==
  "p{4}" : Inport  PortDimensions=10  SampleTime=0.1
      mask Display: e = 0.06;c1 = [120 230 180]/255;c2 = ([120 230 180]+0)/(256+128);c3 = ([120 230 180]+128)/(256+128);patch([0 1 1 0],[0 0 1 1],c1);patch([0 1 1 1-e 1-e 0+e],[0 0 1 1-e 0+e 0+e],c2);patch([0 0 1 1-e 0+e 0+e],[0 1 1 1-e 1-e 0+e],c3);plot([0 1 1 0 0],[0 0 1 1 0]);
  mux : Mux  Inputs=1
      mask Display: e = 0.06;c1 = [120 150 230]/255;c2 = ([120 150 230]+0)/383;c3 = ([120 150 230]+128)/383;patch([0 1 1 0],[0 0 1 1],c1);patch([0 1 1 1-e 1-e 0+e],[0 0 1 1-e 0+e 0+e],c2);patch([0 0 1 1-e 0+e 0+e],[0 1 1 1-e 1-e 0+e],c3);plot([0 1 1 0 0],[0 0 1 1 0]);disp('Mux')
  "pd{4,3}" : Outport
      mask Display: e = 0.06;c1 = [120 230 180]/255;c2 = ([120 230 180]+0)/(256+128);c3 = ([120 230 180]+128)/(256+128);patch([0 1 1 0],[0 0 1 1],c1);patch([0 1 1 1-e 1-e 0+e],[0 0 1 1-e 0+e 0+e],c2);patch([0 0 1 1-e 0+e 0+e],[0 1 1 1-e 1-e 0+e],c3);plot([0 1 1 0 0],[0 0 1 1 0]);
  wires:
  "p{4}"/1 -> mux/1
  mux/1 -> "pd{4,3}"/1

== system ackerman_ROS_neural_controller_v2/casi 2 - no para1/Layer 4/LW{4,3} ==
  "ad{4,3}" : Inport  PortDimensions=10  SampleTime=0.1
      mask Display: e = 0.06;c1 = [120 230 180]/255;c2 = ([120 230 180]+0)/(256+128);c3 = ([120 230 180]+128)/(256+128);patch([0 1 1 0],[0 0 1 1],c1);patch([0 1 1 1-e 1-e 0+e],[0 0 1 1-e 0+e 0+e],c2);patch([0 0 1 1-e 0+e 0+e],[0 1 1 1-e 1-e 0+e],c3);plot([0 1 1 0 0],[0 0 1 1 0]);
  "IW{4,3}(1,:)'" : Constant  Value=[0.86322822727236980799858656610012985765933990478515625;1.7639738025649480679390990189858712255954742431640625;0.85681753345993738602004441418102942407131195068359375;0.66445653674042570724367351431283168494701385498046875;-0.80756424705848728340384923285455442965030670166015625;-0.41632510960593271942542514807428233325481414794921875;-0.98607912436545286372080454384558834135532379150390625;-0.17594677866998209569970867960364557802677154541015625;-0.810264583193305298891573329456150531768798828125;-0.65162545454995324245572874133358709514141082763671875]
      mask Display: e = 0.06;c1 = [120 150 230]/255;c2 = ([120 150 230]+0)/383;c3 = ([120 150 230]+128)/383;patch([0 1 1 0],[0 0 1 1],c1);patch([0 1 1 1-e 1-e 0+e],[0 0 1 1-e 0+e 0+e],c2);patch([0 0 1 1-e 0+e 0+e],[0 1 1 1-e 1-e 0+e],c3);plot([0 1 1 0 0],[0 0 1 1 0]);disp('weights');
  "IW{4,3}(2,:)'" : Constant  Value=[-0.85284869991453959858773714586277492344379425048828125;0.492365087605975748630271482397802174091339111328125;0.85181177918368755630496025332831777632236480712890625;-0.6202415928991953375515322477440349757671356201171875;-0.53035258340782487351816598675213754177093505859375;0.269544294261485017916157858053338713943958282470703125;-0.5697810416809339084664998154039494693279266357421875;-0.3689105198487319103861636904184706509113311767578125;-0.71190071704257251727909761029877699911594390869140625;-0.77598327561900692916907473772880621254444122314453125]
      mask Display: e = 0.06;c1 = [120 150 230]/255;c2 = ([120 150 230]+0)/383;c3 = ([120 150 230]+128)/383;patch([0 1 1 0],[0 0 1 1],c1);patch([0 1 1 1-e 1-e 0+e],[0 0 1 1-e 0+e 0+e],c2);patch([0 0 1 1-e 0+e 0+e],[0 1 1 1-e 1-e 0+e],c3);plot([0 1 1 0 0],[0 0 1 1 0]);disp('weights');
  Mux : Mux  Inputs=2
      mask Display: e = 0.06;c1 = [120 150 230]/255;c2 = ([120 150 230]+0)/383;c3 = ([120 150 230]+128)/383;patch([0 1 1 0],[0 0 1 1],c1);patch([0 1 1 1-e 1-e 0+e],[0 0 1 1-e 0+e 0+e],c2);patch([0 0 1 1-e 0+e 0+e],[0 1 1 1-e 1-e 0+e],c3);plot([0 1 1 0 0],[0 0 1 1 0]);disp('Mux');
  dotprod1 : neural/Weight Functions/dotprod
  dotprod2 : neural/Weight Functions/dotprod
  "lz{4,3}" : Outport
      mask Display: e = 0.06;c1 = [120 230 180]/255;c2 = ([120 230 180]+0)/(256+128);c3 = ([120 230 180]+128)/(256+128);patch([0 1 1 0],[0 0 1 1],c1);patch([0 1 1 1-e 1-e 0+e],[0 0 1 1-e 0+e 0+e],c2);patch([0 0 1 1-e 0+e 0+e],[0 1 1 1-e 1-e 0+e],c3);plot([0 1 1 0 0],[0 0 1 1 0]);
  wires:
  "IW{4,3}(1,:)'"/1 -> dotprod1/1
  "ad{4,3}"/1 -> dotprod1/2, dotprod2/2
  dotprod1/1 -> Mux/1
  "IW{4,3}(2,:)'"/1 -> dotprod2/1
  dotprod2/1 -> Mux/2
  Mux/1 -> "lz{4,3}"/1

== system ackerman_ROS_neural_controller_v2/casi 3 - 15 20 15/Layer 1/Delays 1 ==
  "p{1}" : Inport  PortDimensions=8  SampleTime=0.1
      mask Display: e = 0.06;c1 = [120 230 180]/255;c2 = ([120 230 180]+0)/(256+128);c3 = ([120 230 180]+128)/(256+128);patch([0 1 1 0],[0 0 1 1],c1);patch([0 1 1 1-e 1-e 0+e],[0 0 1 1-e 0+e 0+e],c2);patch([0 0 1 1-e 0+e 0+e],[0 1 1 1-e 1-e 0+e],c3);plot([0 1 1 0 0],[0 0 1 1 0]);
  mux : Mux  Inputs=1
      mask Display: e = 0.06;c1 = [120 150 230]/255;c2 = ([120 150 230]+0)/383;c3 = ([120 150 230]+128)/383;patch([0 1 1 0],[0 0 1 1],c1);patch([0 1 1 1-e 1-e 0+e],[0 0 1 1-e 0+e 0+e],c2);patch([0 0 1 1-e 0+e 0+e],[0 1 1 1-e 1-e 0+e],c3);plot([0 1 1 0 0],[0 0 1 1 0]);disp('Mux')
  "pd{1,1}" : Outport
      mask Display: e = 0.06;c1 = [120 230 180]/255;c2 = ([120 230 180]+0)/(256+128);c3 = ([120 230 180]+128)/(256+128);patch([0 1 1 0],[0 0 1 1],c1);patch([0 1 1 1-e 1-e 0+e],[0 0 1 1-e 0+e 0+e],c2);patch([0 0 1 1-e 0+e 0+e],[0 1 1 1-e 1-e 0+e],c3);plot([0 1 1 0 0],[0 0 1 1 0]);
  wires:
  "p{1}"/1 -> mux/1
  mux/1 -> "pd{1,1}"/1
